simulink model "lfc2AreaWithoutController"  (R2024a)
settings: Solver=VariableStepAuto  StartTime=0.0  StopTime=20  RelTol=1e-3
settings Model: Creator=farza  LastModifiedBy=farza

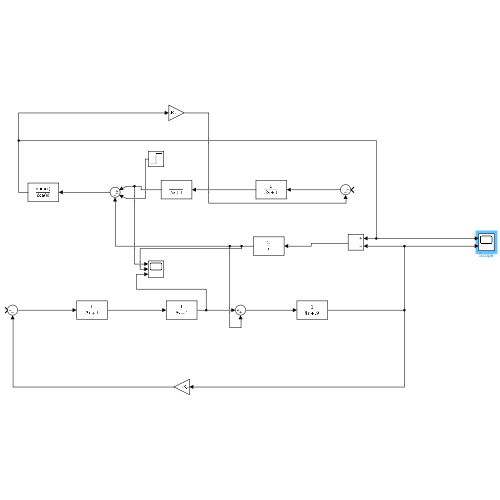
[thumbnail: Simulink's stored preview of the top-level diagram]
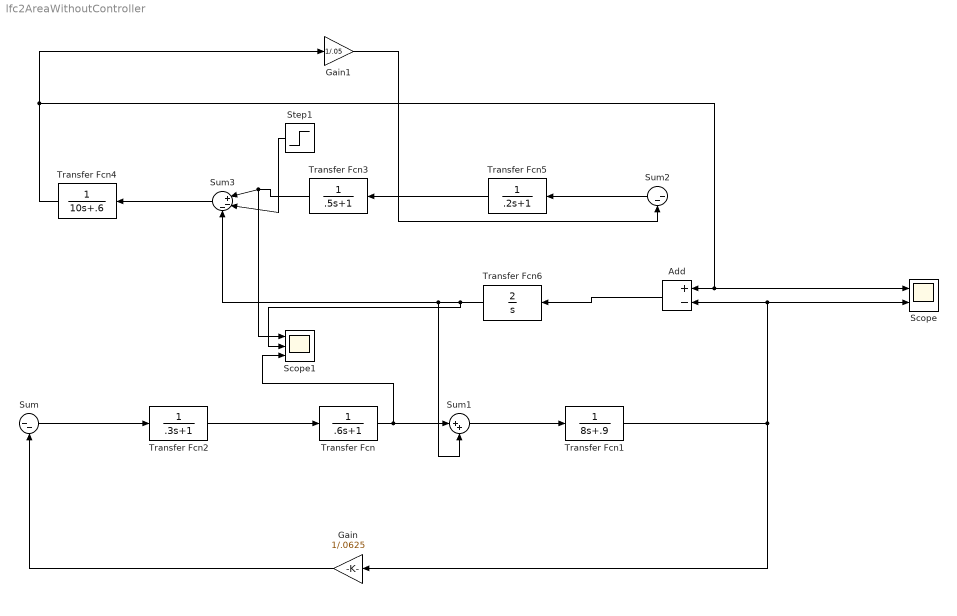
== system lfc2AreaWithoutController ==
  Add : Sum  Inputs=+-
  Gain : Gain  Gain=1/.0625
  Gain1 : Gain  Gain=1/.05
  Scope : Scope  NumInputPorts=2
  Scope1 : Scope  NumInputPorts=3
  Step1 : Step  After=.2  SampleTime=0
  Sum : Sum  Inputs=|--
  Sum1 : Sum  Inputs=|++
  Sum2 : Sum  Inputs=|--
  Sum3 : Sum  Inputs=|+--
  Transfer Fcn : TransferFcn  Denominator=[.6 1]
  Transfer Fcn1 : TransferFcn  Denominator=[8 .9]
  Transfer Fcn2 : TransferFcn  Denominator=[.3 1]
  Transfer Fcn3 : TransferFcn  Denominator=[.5 1]
  Transfer Fcn4 : TransferFcn  Denominator=[10 .6]
  Transfer Fcn5 : TransferFcn  Denominator=[.2 1]
  Transfer Fcn6 : TransferFcn  Numerator=2  Denominator=[1 0]
  wires:
  Sum/1 -> Transfer Fcn2/1
  Transfer Fcn2/1 -> Transfer Fcn/1
  Transfer Fcn/1 -> Scope1/3, Sum1/1
  Sum1/1 -> Transfer Fcn1/1
  Transfer Fcn1/1 -> Scope/2, Add/2, Gain/1
  Gain/1 -> Sum/2
  Gain1/1 -> Sum2/2
  Sum3/1 -> Transfer Fcn4/1
  Step1/1 -> Sum3/2
  Transfer Fcn5/1 -> Transfer Fcn3/1
  Transfer Fcn4/1 -> Scope/1, Add/1, Gain1/1
  Transfer Fcn3/1 -> Scope1/1, Sum3/1
  Sum2/1 -> Transfer Fcn5/1
  Transfer Fcn6/1 -> Scope1/2, Sum1/2, Sum3/3
  Add/1 -> Transfer Fcn6/1
